simulink model "kalmanfilter2"  (Simulink 6.5)
settings: Solver=ode1  StartTime=0.0  StopTime=10  FixedStep=0.001  RelTol=1e-3
settings Model: Creator=fo1521  LastModifiedBy=Jskb
settings DebuggingCC: SignalResolutionControl=UseLocalSettings  MultiTaskCondExecSysMsg=none  StrictBusMsg=None
settings HardwareCC: TargetHWDeviceType=32-bit Generic
settings RTWCC: IncludeERTFirstTime=on

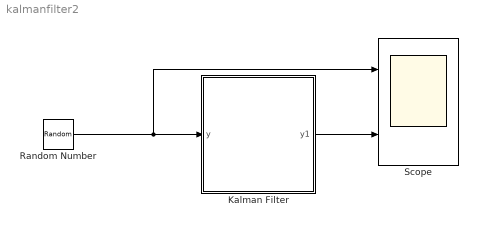
== system kalmanfilter2 ==
  Kalman Filter : Subsystem  mask{x0=0, P0=1000, A=1, B=0, C=1, D=0, Q=0.01, R=10}
      mask help:
      | Linear Random Process
      | x(k+1)=Ax(k)+Bu(k)+w
      | y(k)=Cx(k)+Du(k)+v
      | w~N(0,Q)
      | w~N(0,R)
  Random Number : RandomNumber  Mean=10  Variance=10  SampleTime=0
  Scope : Scope  NumInputPorts=2
      settings: TimeRange=10  YMin=-20~8  YMax=40~14
  wires:
  Random Number/1 -> Kalman Filter/1(y), Scope/1
  Kalman Filter/1(y1) -> Scope/2

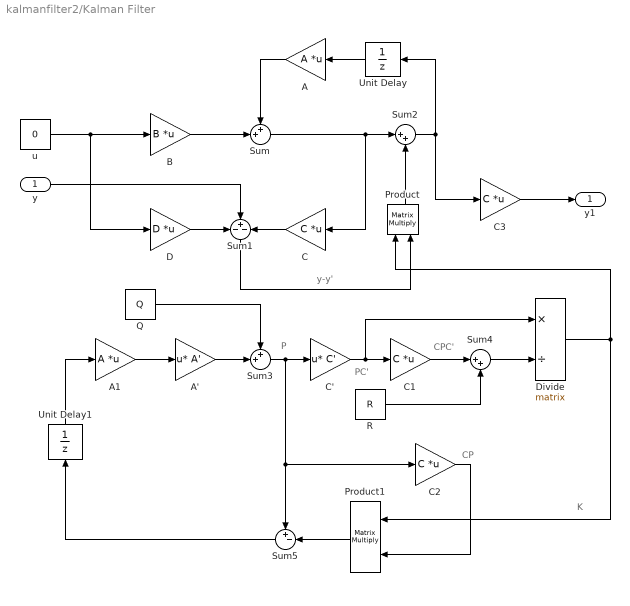
== system kalmanfilter2/Kalman Filter ==
  note: P
  note: PC'
  note: CPC'
  note: K
  note: CP
  note: y-y'
  y : Inport
  A : Gain  Orientation=left  Gain=A  Multiplication=Matrix(K*u)
  A' : Gain  Gain=A'  Multiplication=Matrix(u*K)
  A1 : Gain  Gain=A  Multiplication=Matrix(K*u)
  B : Gain  Gain=B  Multiplication=Matrix(K*u)
  C : Gain  Orientation=left  Gain=C  Multiplication=Matrix(K*u)
  C' : Gain  Gain=C'  Multiplication=Matrix(u*K)
  C1 : Gain  Gain=C  Multiplication=Matrix(K*u)
  C2 : Gain  Gain=C  Multiplication=Matrix(K*u)
  C3 : Gain  Gain=C  Multiplication=Matrix(K*u)
  D : Gain  Gain=D  Multiplication=Matrix(K*u)
  Divide : Product  Inputs=*/  Multiplication=Matrix(*)  OutScaling=2^-10
  Product : Product  Orientation=up  Multiplication=Matrix(*)  RndMeth=Zero
  Product1 : Product  Orientation=left  Multiplication=Matrix(*)  RndMeth=Zero
  Q : Constant  Value=Q  OutDataType=sfix(16)  ConRadixGroup=Use specified scaling  OutScaling=2^0  SampleTime=inf  FramePeriod=inf
  R : Constant  Value=R  OutDataType=sfix(16)  ConRadixGroup=Use specified scaling  OutScaling=2^0  SampleTime=inf  FramePeriod=inf
  Sum : Sum  Inputs=++|
  Sum1 : Sum  Orientation=down  Inputs=-+-
  Sum2 : Sum  Inputs=|++
  Sum3 : Sum  Inputs=++|
  Sum4 : Sum  Inputs=|++
  Sum5 : Sum  Orientation=left  Inputs=+-|
  Unit Delay : UnitDelay  Orientation=left  X0=x0  SampleTime=-1
  Unit Delay1 : UnitDelay  Orientation=up  X0=P0  SampleTime=-1
  u : Constant  Value=0  OutDataType=sfix(16)  ConRadixGroup=Use specified scaling  OutScaling=2^0  SampleTime=inf  FramePeriod=inf
  y1 : Outport
  wires:
  u/1 -> B/1, D/1
  B/1 -> Sum/2
  A/1 -> Sum/1
  Unit Delay/1 -> A/1
  Sum/1 -> Sum2/1, C/1
  Sum2/1 -> Unit Delay/1, C3/1
  D/1 -> Sum1/1
  C/1 -> Sum1/3
  y/1 -> Sum1/2
  A1/1 -> A'/1
  A'/1 -> Sum3/2
  Q/1 -> Sum3/1
  Sum3/1 -> C'/1, Sum5/1, C2/1
  C'/1 -> C1/1, Divide/1
  Product/1 -> Sum2/2
  Divide/1 -> Product/1, Product1/1
  Product1/1 -> Sum5/2
  C1/1 -> Sum4/1
  R/1 -> Sum4/2
  Sum4/1 -> Divide/2
  Unit Delay1/1 -> A1/1
  Sum5/1 -> Unit Delay1/1
  C3/1 -> y1/1
  Sum1/1 -> Product/2
  C2/1 -> Product1/2
